simulink model "basic_04_robot"  (R2016a)
settings: Solver=FixedStepAuto  StartTime=0.0  StopTime=inf  FixedStep=0.001  RelTol=1e-3
libraries: Robot_ToolBox x20
settings Model: SimulationMode=external  Creator=Wang Yifan  LastModifiedBy=Wang Yifan
settings OptimizationCC: OptimizeModelRefInitCode=on  LifeSpan=Inf
settings HardwareCC: ProdBitPerLong=64  ProdHWDeviceType=Intel->x86-64 (Linux 64)  TargetBitPerLong=64  TargetBitPerPointer=64  TargetLargestAtomicFloat=Float  TargetIntDivRoundTo=Zero  TargetEndianess=LittleEndian  TargetWordSize=64  TargetHWDeviceType=Intel->x86-64 (Linux 64)  ProdEqTarget=off
settings RTWCC: SystemTargetFile=linux_ert_target.tlc  GenCodeOnly=on  MakeCommand=make_rtw CC=gcc  TemplateMakefile=linux_ert_target.tmf  Description=Linux Embedded Real-Time target  RetainRTWFile=on
settings CodeAppCC: ForceParamTrailComments=on  IgnoreCustomStorageClasses=off  OperatorAnnotations=on  SimulinkDataObjDesc=on  SFDataObjDesc=on  MATLABFcnDesc=on  InsertBlockDesc=on  MATLABSourceComments=on
settings STFCustomTargetCC: CombineOutputUpdateFcns=on  ERTCustomFileBanners=on  SupportContinuousTime=off  SupportNonInlinedSFcns=off  MATLABClassNameForMDSCustomization=Simulink.SoftwareTarget.ERTCustomization  GRTInterface=off  SystemTargetFile=linux_ert_target.tlc
settings ERTTargetCC: ParMdlRefBuildCompliant=off  CompOptLevelCompliant=off  ConcurrentExecutionCompliant=off  ERTFirstTimeCompliant=off  ModelStepFunctionPrototypeControlCompliant=off  CPPClassGenCompliant=off  UseToolchainInfoCompliant=off  ExtMode=on  ExtModeMexArgs='192.168.0.99' 1 17725  ERTSrcFileBannerTemplate=linux_ert_target_code_template.cgt  ERTHdrFileBannerTemplate=linux_ert_target_code_template.cgt  ERTDataSrcFileTemplate=linux_ert_target_code_template.cgt  ERTDataHdrFileTemplate=linux_ert_target_code_template.cgt  ERTCustomFileTemplate=linux_ert_target_generate_main.tlc

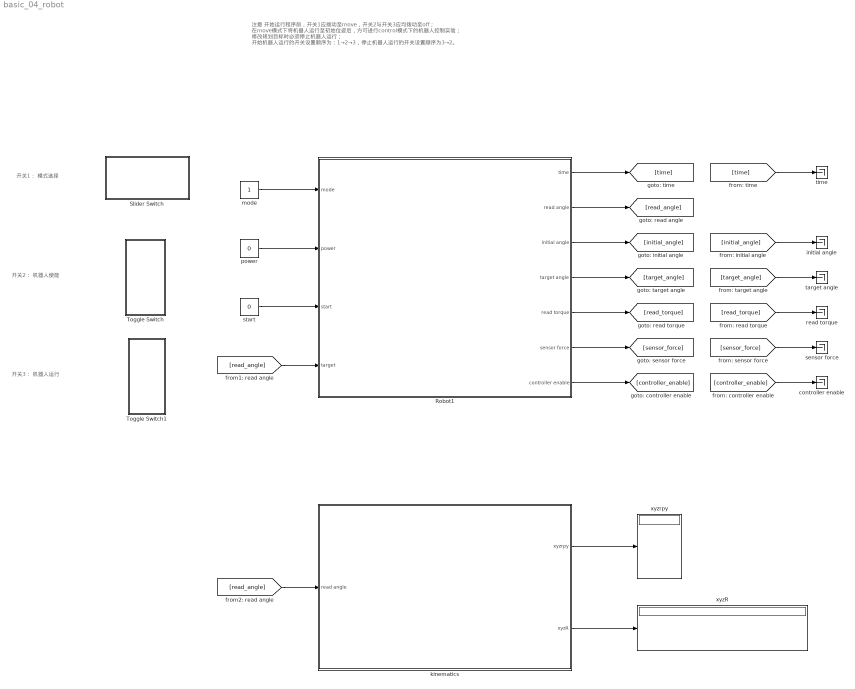
== system basic_04_robot ==
  note: 开关3： 机器人运行
  note: 开关1： 模式选择
  note: 开关2： 机器人使能
  note: 注意
      |
      | 开始运行程序前，开关1应拨动至move，开关2与开关3应均拨动至off；
      | 在move模式下将机器人运行至初始位姿后，方可进行control模式下的机器人控制实验；
      | 修改规划目标时必须停止机器人运行；
      | 开始机器人运行的开关设置顺序为：1→2→3，停止机器人运行的开关设置顺序为3→2。
  Robot1 : Subsystem  mask{move_joint=[0 0 0 0 0 0], joint_1_limit=[-pi/2, pi/2], joint_2_limit=[-pi/2, pi/2], joint_3_limit=[-pi/2, pi/2], joint_4_limit=[-pi/2, pi/2], joint_5_limit=[-pi/2, pi/2], joint_6_limit=[-pi/2, pi/2]}
      mask prompts: joint_1_limit "Joint 1"; joint_2_limit "Joint 2"; joint_3_limit "Joint 3"; joint_4_limit "Joint 4"; joint_5_limit "Joint 5"; joint_6_limit "Joint 6"
      mask DialogControl Container1 Prompt: 目标关节角(rad)
      mask DialogControl Control1 Prompt: e.g. [0 0 0 0 0 0]
      mask DialogControl Container2 Prompt: 关节限位(rad)
      mask DialogControl Control2 Prompt: e.g. [-pi/2, pi/2]
      mask DialogControl Container3 Prompt: 注意：不需要对此模块内部进行修改
  Slider Switch : Subsystem  DialogController=hmiCreateDDGDialog  IsWebBlock=on  mask(MWDashboardBlock){webBlockId=826f4840-ab60-43d7-9b3b-f5102fb9e134, webBlockType=sliderswitch, ShowInLibBrowser=on, ShowInitialText=on, HMISrcModelName=basic_04_robot}
      mask prompts: webBlockId "WebBlock Id"; webBlockType "WebBlock Type"; HMISrcModelName "Source Model"
      mask Help: helpview([docroot '/mapfiles/simulink.map'], 'hmi_slider_switch')
      mask Display:
      | if strcmp(get_param(bdroot(gcb),'BlockDiagramType'), 'library')
      |     image([(matlabroot) '/toolbox/simulink/hmi/icons/SliderSwitch.png']);
      | end
  Toggle Switch : Subsystem  DialogController=hmiCreateDDGDialog  IsWebBlock=on  mask(MWDashboardBlock){webBlockId=da419e04-a9a7-4766-8422-35a2c91d1971, webBlockType=toggleswitch, ShowInLibBrowser=on, ShowInitialText=on, HMISrcModelName=basic_04_robot}
      mask prompts: webBlockId "WebBlock Id"; webBlockType "WebBlock Type"; HMISrcModelName "Source Model"
      mask Help: helpview([docroot '/mapfiles/simulink.map'], 'hmi_toggle_switch')
      mask Display:
      | if strcmp(get_param(bdroot(gcb),'BlockDiagramType'), 'library')
      |     image([(matlabroot) '/toolbox/simulink/hmi/icons/ToggleSwitch.png']);
      | end
  Toggle Switch1 : Subsystem  DialogController=hmiCreateDDGDialog  IsWebBlock=on  mask(MWDashboardBlock){webBlockId=ca3441fb-96d4-41d4-ba82-c21ec3149ad6, webBlockType=toggleswitch, ShowInLibBrowser=on, ShowInitialText=on, HMISrcModelName=basic_04_robot}
      mask prompts: webBlockId "WebBlock Id"; webBlockType "WebBlock Type"; HMISrcModelName "Source Model"
      mask Help: helpview([docroot '/mapfiles/simulink.map'], 'hmi_toggle_switch')
      mask Display:
      | if strcmp(get_param(bdroot(gcb),'BlockDiagramType'), 'library')
      |     image([(matlabroot) '/toolbox/simulink/hmi/icons/ToggleSwitch.png']);
      | end
  controller enable : Terminator
  initial angle : Terminator
  kinematics : Subsystem
  mode : Constant
  power : Constant  Value=0
  read torque : Terminator
  sensor force : Terminator
  start : Constant  Value=0
  target angle : Terminator
  time : Terminator
  xyzR : Display
      settings: Decimation=6
  xyzrpy : Display
      settings: Decimation=6
  wires:
  mode/1 -> Robot1/1(mode)
  power/1 -> Robot1/2(power)
  Robot1/2(read angle) -> [read_angle]
  Robot1/1(time) -> [time]
  Robot1/7(controller enable) -> [controller_enable]
  Robot1/4(target angle) -> [target_angle]
  Robot1/6(sensor force) -> [sensor_force]
  Robot1/3(initial angle) -> [initial_angle]
  start/1 -> Robot1/3(start)
  Robot1/5(read torque) -> [read_torque]
  [time] -> time/1
  [read_angle] -> kinematics/1(read angle)
  [initial_angle] -> initial angle/1
  [target_angle] -> target angle/1
  [read_torque] -> read torque/1
  [sensor_force] -> sensor force/1
  [controller_enable] -> controller enable/1
  kinematics/1(xyzrpy) -> xyzrpy/1
  kinematics/2(xyzR) -> xyzR/1
  [read_angle] -> Robot1/4(target)

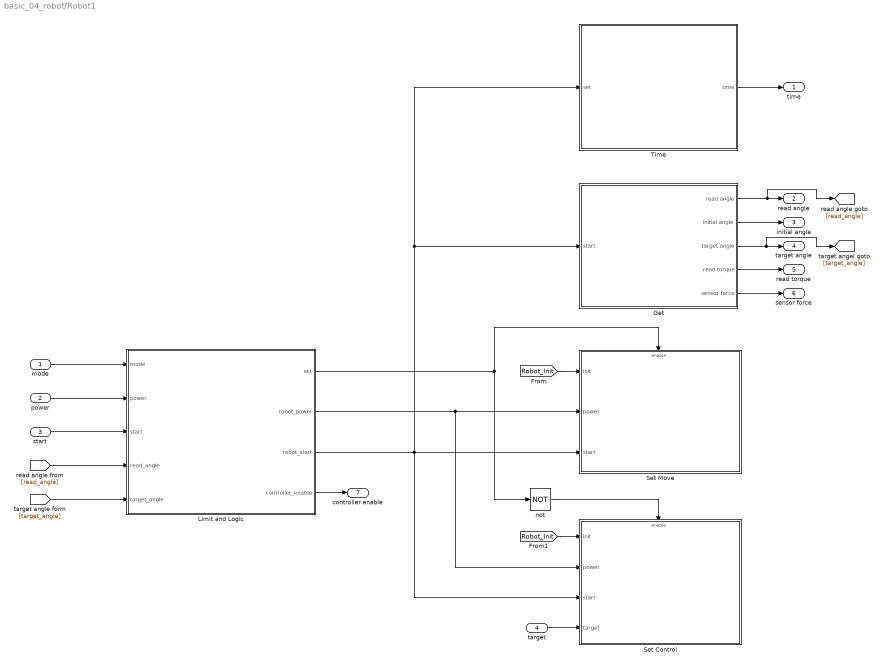
== system basic_04_robot/Robot1 ==
  mode : Inport
  power : Inport  Port=2
  start : Inport  Port=3
  target : Inport  Port=4
  Get : Subsystem
  Limit and Logic : Subsystem
  Set Control : Subsystem  mask(机器人控制模式){mode=Position Mode}
      mask prompts: mode "Control Mode"
      mask TypeOptions mode: Position Mode | Torque Mode | Velocity Mode
  Set Move : Subsystem
  Time : Subsystem
  not : Logic  Operator=NOT  AllPortsSameDT=off  OutDataTypeStr=boolean
  time : Outport
  read angle : Outport  Port=2
  initial angle : Outport  Port=3
  target angle : Outport  Port=4
  read torque : Outport  Port=5
  sensor force : Outport  Port=6
  controller enable : Outport  Port=7
  wires:
  target/1 -> Set Control/4(target)
  Get/1(read angle) -> [read_angle], read angle/1
  Time/1(time) -> time/1
  Get/2(initial angle) -> initial angle/1
  Get/3(target angle) -> [target_angle], target angle/1
  Get/5(sensor force) -> sensor force/1
  Limit and Logic/1(set) -> Set Move/Enable, not/1
  not/1 -> Set Control/Enable
  Limit and Logic/2(robot_power) -> Set Control/2(power), Set Move/2(power)
  Limit and Logic/4(controller_enable) -> controller enable/1
  Limit and Logic/3(robot_start) -> Set Control/3(start), Set Move/3(start), Time/1(set), Get/1(start)
  [Robot_Init] -> Set Move/1(init)
  [Robot_Init] -> Set Control/1(init)
  Get/4(read torque) -> read torque/1
  mode/1 -> Limit and Logic/1(mode)
  power/1 -> Limit and Logic/2(power)
  start/1 -> Limit and Logic/3(start)
  [read_angle] -> Limit and Logic/4(read_angle)
  [target_angle] -> Limit and Logic/5(target_angle)

== system basic_04_robot/Slider Switch ==

== system basic_04_robot/Toggle Switch ==

== system basic_04_robot/Toggle Switch1 ==

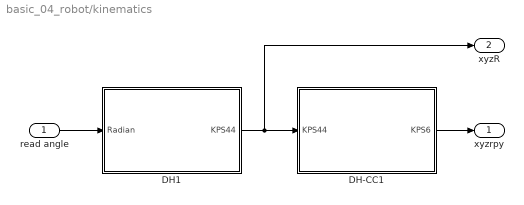
== system basic_04_robot/kinematics ==
  read angle : Inport
  DH-CC1 : MATLAB Function  TreatAsAtomicUnit=on
  DH1 : MATLAB Function  TreatAsAtomicUnit=on
  xyzrpy : Outport
  xyzR : Outport  Port=2
  wires:
  DH1/1(KPS44) -> xyzR/1, DH-CC1/1(KPS44)
  read angle/1 -> DH1/1(Radian)
  DH-CC1/1(KPS6) -> xyzrpy/1

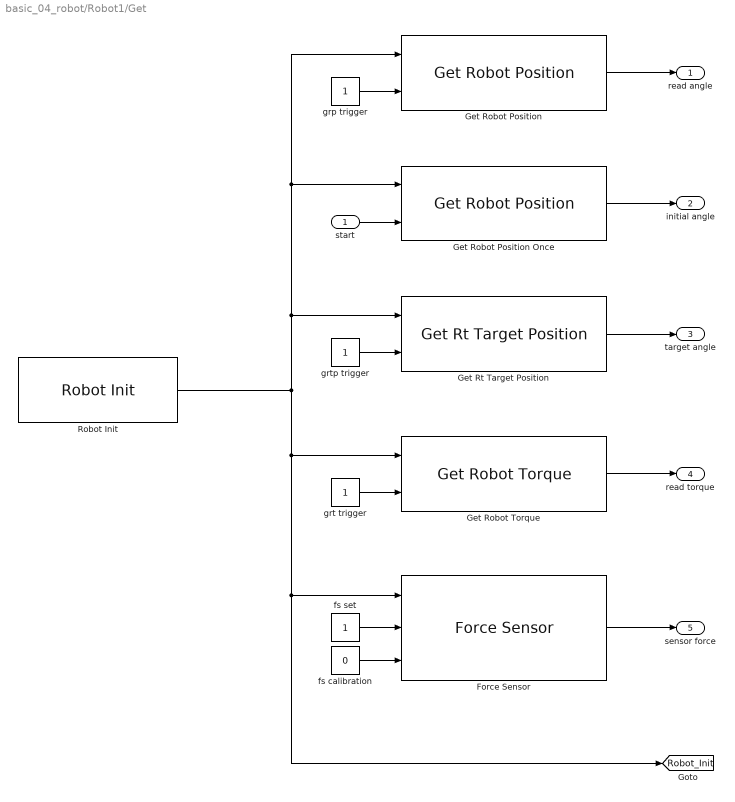
== system basic_04_robot/Robot1/Get ==
  start : Inport
  Force Sensor : Robot_ToolBox/Sensor/Force Sensor  p_robot_index=0  p_torsensor_index=0  p_tool=0  p_wobj=0  p_system_tor_flag=off  p_transform_flag=on
  Get Robot Position : Robot_ToolBox/Robot Interface/Get Robot Position  p_robot_index=0  p_block_index=1  p_read_once=off
  Get Robot Position Once : Robot_ToolBox/Robot Interface/Get Robot Position  p_robot_index=0  p_block_index=0  p_read_once=on
  Get Robot Torque : Robot_ToolBox/Robot Interface/Get Robot Torque  p_robot_index=0  p_block_index=0  p_read_once=off
  Get Rt Target Position : Robot_ToolBox/Robot Interface/Get Rt Target Position  p_robot_index=0  p_block_index=0  p_read_once=off
  Robot Init : Robot_ToolBox/Robot System Tool/Robot Init
  fs calibration : Constant  Value=0
  fs set : Constant
  grp trigger : Constant
  grt trigger : Constant
  grtp trigger : Constant
  read angle : Outport
  initial angle : Outport  Port=2
  target angle : Outport  Port=3
  read torque : Outport  Port=4
  sensor force : Outport  Port=5
  tag scope: Robot_Init=global
  wires:
  Robot Init/1 -> Get Robot Position/1, Get Robot Position Once/1, Get Rt Target Position/1, [Robot_Init], Force Sensor/1, Get Robot Torque/1
  Get Robot Position/1 -> read angle/1
  Get Robot Position Once/1 -> initial angle/1
  Get Rt Target Position/1 -> target angle/1
  Force Sensor/1 -> sensor force/1
  grp trigger/1 -> Get Robot Position/2
  grtp trigger/1 -> Get Rt Target Position/2
  fs set/1 -> Force Sensor/2
  fs calibration/1 -> Force Sensor/3
  start/1 -> Get Robot Position Once/2
  grt trigger/1 -> Get Robot Torque/2
  Get Robot Torque/1 -> read torque/1

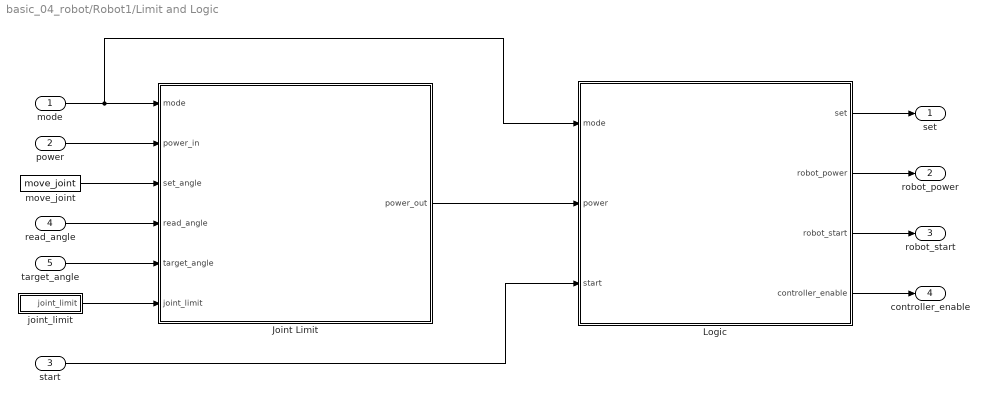
== system basic_04_robot/Robot1/Limit and Logic ==
  mode : Inport
  power : Inport  Port=2
  start : Inport  Port=3
  read_angle : Inport  Port=4
  target_angle : Inport  Port=5
  Joint Limit : MATLAB Function  TreatAsAtomicUnit=on
  Logic : Stateflow chart  TreatAsAtomicUnit=on
  joint_limit : Subsystem
  move_joint : Constant  Value=move_joint
  set : Outport
  robot_power : Outport  Port=2
  robot_start : Outport  Port=3
  controller_enable : Outport  Port=4
  wires:
  Joint Limit/1(power_out) -> Logic/2(power)
  read_angle/1 -> Joint Limit/4(read_angle)
  target_angle/1 -> Joint Limit/5(target_angle)
  mode/1 -> Logic/1(mode), Joint Limit/1(mode)
  power/1 -> Joint Limit/2(power_in)
  start/1 -> Logic/3(start)
  Logic/1(set) -> set/1
  Logic/2(robot_power) -> robot_power/1
  Logic/3(robot_start) -> robot_start/1
  Logic/4(controller_enable) -> controller_enable/1
  move_joint/1 -> Joint Limit/3(set_angle)
  joint_limit/1(joint_limit) -> Joint Limit/6(joint_limit)

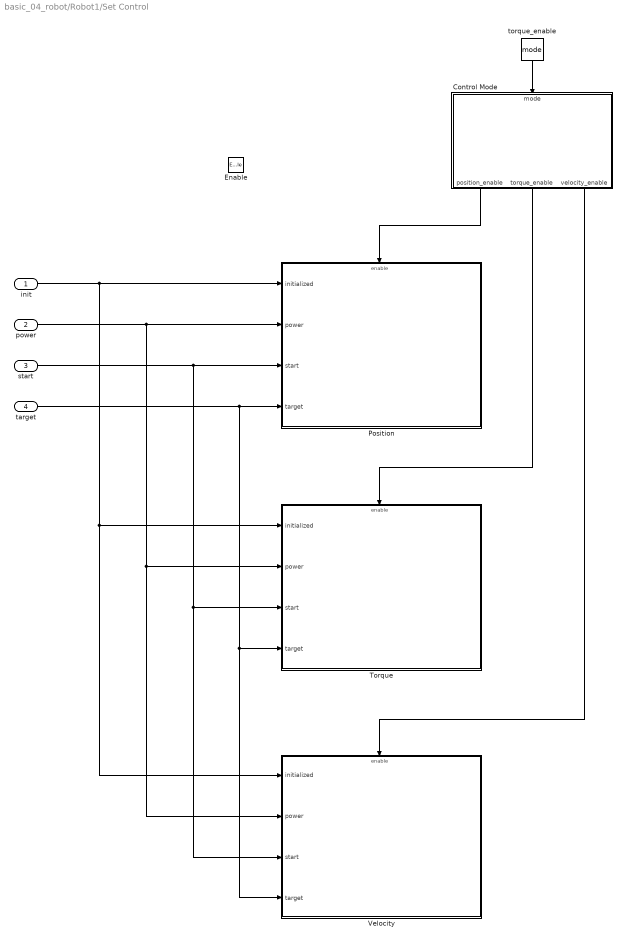
== system basic_04_robot/Robot1/Set Control ==
  init : Inport
  power : Inport  Port=2
  start : Inport  Port=3
  target : Inport  Port=4
  Enable : EnablePort
  Control Mode : Stateflow chart  TreatAsAtomicUnit=on
  Position : Subsystem
  Torque : Subsystem
  Velocity : Subsystem
  torque_enable : Constant  Value=mode
  wires:
  init/1 -> Position/1(initialized), Velocity/1(initialized), Torque/1(initialized)
  power/1 -> Velocity/2(power), Torque/2(power), Position/2(power)
  start/1 -> Velocity/3(start), Torque/3(start), Position/3(start)
  target/1 -> Velocity/4(target), Torque/4(target), Position/4(target)
  Control Mode/1(position_enable) -> Position/Enable
  torque_enable/1 -> Control Mode/1(mode)
  Control Mode/2(torque_enable) -> Torque/Enable
  Control Mode/3(velocity_enable) -> Velocity/Enable

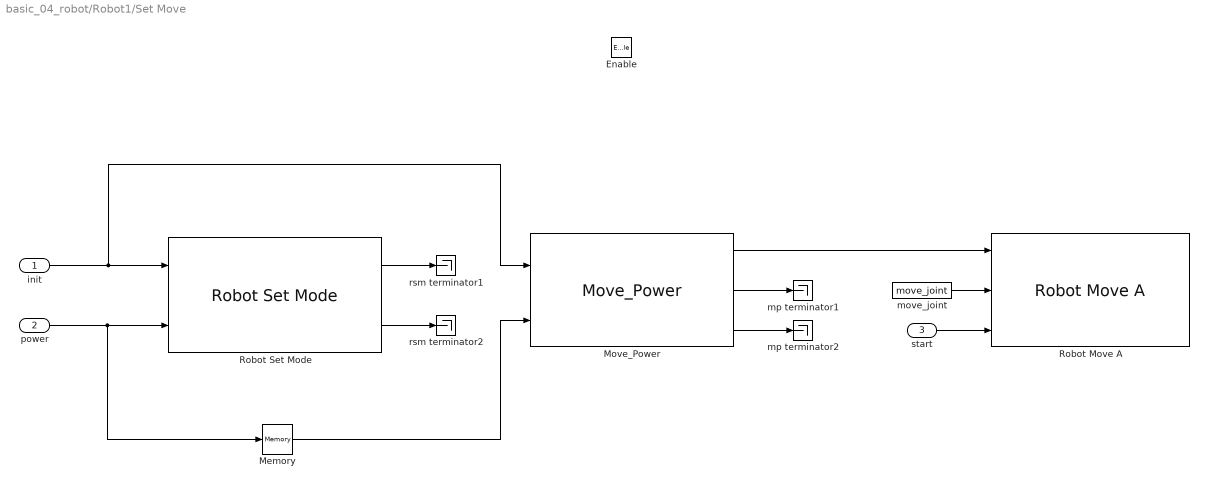
== system basic_04_robot/Robot1/Set Move ==
  init : Inport
  power : Inport  Port=2
  start : Inport  Port=3
  Enable : EnablePort
  Memory : Memory
  Move_Power : Robot_ToolBox/Robot Base Conrtrol/Move_Power  p_robot_index=0  p_block_index=0
      link override S-Function Builder: Parameters=p_robot_index,p_block_index,p_move_thread
  Robot Move A : Robot_ToolBox/Robot Base Conrtrol/Robot Move A  p_robot_index=0  p_block_index=0  p_MoveA_per=[10 10 10 10 10 10]  p_MoveA_per_flag=2  p_zone=0  p_tool=0  p_wobj=0
      link override MoveA: Parameters=p_robot_index,p_block_index,p_MoveA_per,int32(p_MoveA_per_flag),p_zone,p_tool,p_wobj
  Robot Set Mode : Robot_ToolBox/Robot System Tool/Robot Set Mode  p_robot_index=0  p_block_index=0  p_robot_mode=位置模式  p_robot_all=on  p_robot_Axis1=on  p_robot_Axis2=on  p_robot_Axis3=on  p_robot_Axis4=on  p_robot_Axis5=on  p_robot_Axis6=on  p_robot_Axis_add=off
  move_joint : Constant  Value=move_joint
  mp terminator1 : Terminator
  mp terminator2 : Terminator
  rsm terminator1 : Terminator
  rsm terminator2 : Terminator
  wires:
  Move_Power/1 -> Robot Move A/1
  move_joint/1 -> Robot Move A/2
  Move_Power/2 -> mp terminator1/1
  Move_Power/3 -> mp terminator2/1
  start/1 -> Robot Move A/3
  power/1 -> Robot Set Mode/2, Memory/1
  Robot Set Mode/1 -> rsm terminator1/1
  Memory/1 -> Move_Power/2
  Robot Set Mode/2 -> rsm terminator2/1
  init/1 -> Move_Power/1, Robot Set Mode/1

== system basic_04_robot/Robot1/Time ==
  set : Inport
  MATLAB Function : MATLAB Function  TreatAsAtomicUnit=on
  Memory : Memory
  time : Outport
  wires:
  set/1 -> MATLAB Function/1(set)
  MATLAB Function/1(t_out) -> time/1, Memory/1
  Memory/1 -> MATLAB Function/2(t_in)

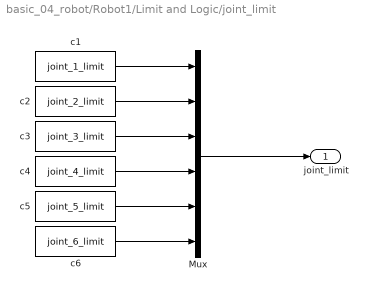
== system basic_04_robot/Robot1/Limit and Logic/joint_limit ==
  Mux : Mux  Inputs=6
  c1 : Constant  Value=joint_1_limit
  c2 : Constant  Value=joint_2_limit
  c3 : Constant  Value=joint_3_limit
  c4 : Constant  Value=joint_4_limit
  c5 : Constant  Value=joint_5_limit
  c6 : Constant  Value=joint_6_limit
  joint_limit : Outport
  wires:
  c1/1 -> Mux/1
  c2/1 -> Mux/2
  c3/1 -> Mux/3
  c4/1 -> Mux/4
  c5/1 -> Mux/5
  c6/1 -> Mux/6
  Mux/1 -> joint_limit/1

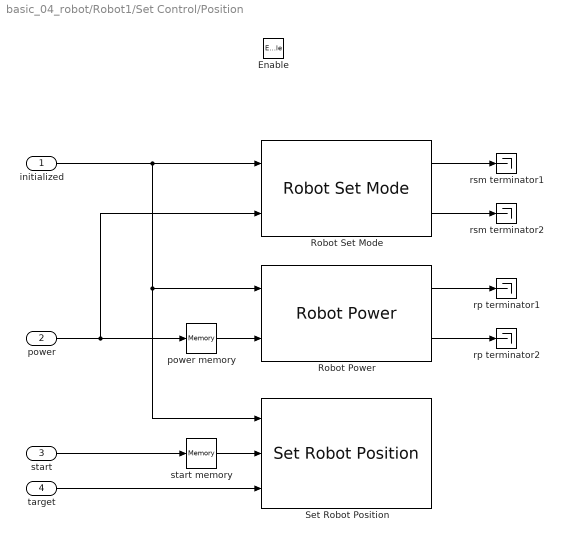
== system basic_04_robot/Robot1/Set Control/Position ==
  initialized : Inport
  power : Inport  Port=2
  start : Inport  Port=3
  target : Inport  Port=4
  Enable : EnablePort
  Robot Power : Robot_ToolBox/Robot System Tool/Robot Power  p_robot_index=0  p_block_index=0  p_robot_all=on  p_robot_Axis1=on  p_robot_Axis2=on  p_robot_Axis3=on  p_robot_Axis4=on  p_robot_Axis5=on  p_robot_Axis6=on  p_robot_Axis_add=off
  Robot Set Mode : Robot_ToolBox/Robot System Tool/Robot Set Mode  p_robot_index=0  p_block_index=0  p_robot_mode=位置模式  p_robot_all=on  p_robot_Axis1=on  p_robot_Axis2=on  p_robot_Axis3=on  p_robot_Axis4=on  p_robot_Axis5=on  p_robot_Axis6=on  p_robot_Axis_add=off
  Set Robot Position : Robot_ToolBox/Robot Interface/Set Robot Position  p_robot_index=0  p_block_index=0  p_read_once=off
  power memory : Memory
  rp terminator1 : Terminator
  rp terminator2 : Terminator
  rsm terminator1 : Terminator
  rsm terminator2 : Terminator
  start memory : Memory
  wires:
  Robot Set Mode/1 -> rsm terminator1/1
  Robot Set Mode/2 -> rsm terminator2/1
  Robot Power/2 -> rp terminator2/1
  initialized/1 -> Robot Set Mode/1, Robot Power/1, Set Robot Position/1
  target/1 -> Set Robot Position/3
  Robot Power/1 -> rp terminator1/1
  power/1 -> power memory/1, Robot Set Mode/2
  start memory/1 -> Set Robot Position/2
  start/1 -> start memory/1
  power memory/1 -> Robot Power/2

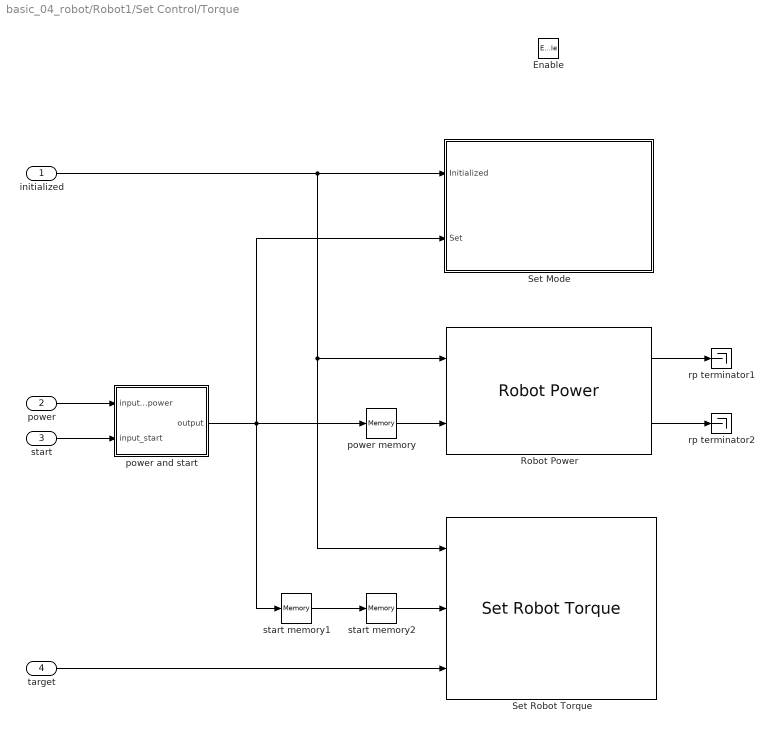
== system basic_04_robot/Robot1/Set Control/Torque ==
  initialized : Inport
  power : Inport  Port=2
  start : Inport  Port=3
  target : Inport  Port=4
  Enable : EnablePort
  Robot Power : Robot_ToolBox/Robot System Tool/Robot Power  p_robot_index=0  p_block_index=0  p_robot_all=off  p_robot_Axis1=off  p_robot_Axis2=off  p_robot_Axis3=off  p_robot_Axis4=off  p_robot_Axis5=off  p_robot_Axis6=on  p_robot_Axis_add=off
  Set Mode : Subsystem
  Set Robot Torque : Robot_ToolBox/Robot Interface/Set Robot Torque  p_robot_index=0  p_block_index=0  p_read_once=off
      link override Set Robot Torque: Parameters=p_robot_index,p_block_index,p_read_once
  power and start : MATLAB Function  TreatAsAtomicUnit=on
  power memory : Memory
  rp terminator1 : Terminator
  rp terminator2 : Terminator
  start memory1 : Memory
  start memory2 : Memory
  wires:
  target/1 -> Set Robot Torque/3
  start memory1/1 -> start memory2/1
  Robot Power/2 -> rp terminator2/1
  Robot Power/1 -> rp terminator1/1
  start memory2/1 -> Set Robot Torque/2
  power memory/1 -> Robot Power/2
  power/1 -> power and start/1(input_power)
  start/1 -> power and start/2(input_start)
  power and start/1(output) -> start memory1/1, Set Mode/2(Set), power memory/1
  initialized/1 -> Robot Power/1, Set Robot Torque/1, Set Mode/1(Initialized)

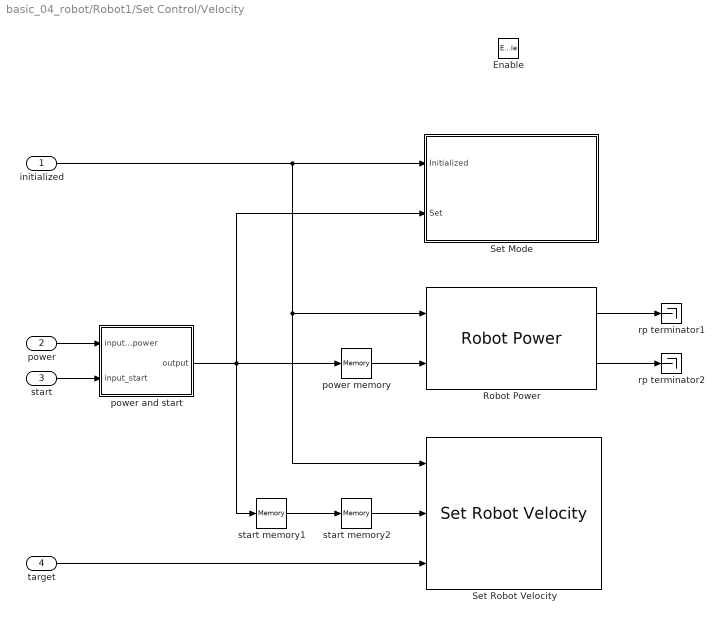
== system basic_04_robot/Robot1/Set Control/Velocity ==
  initialized : Inport
  power : Inport  Port=2
  start : Inport  Port=3
  target : Inport  Port=4
  Enable : EnablePort
  Robot Power : Robot_ToolBox/Robot System Tool/Robot Power  p_robot_index=0  p_block_index=0  p_robot_all=on  p_robot_Axis1=on  p_robot_Axis2=on  p_robot_Axis3=on  p_robot_Axis4=on  p_robot_Axis5=on  p_robot_Axis6=on  p_robot_Axis_add=off
  Set Mode : Subsystem
  Set Robot Velocity : Robot_ToolBox/Robot Interface/Set Robot Velocity  p_robot_index=0  p_block_index=0  p_read_once=off
  power and start : MATLAB Function  TreatAsAtomicUnit=on
  power memory : Memory
  rp terminator1 : Terminator
  rp terminator2 : Terminator
  start memory1 : Memory
  start memory2 : Memory
  wires:
  start memory1/1 -> start memory2/1
  Robot Power/2 -> rp terminator2/1
  Robot Power/1 -> rp terminator1/1
  initialized/1 -> Set Mode/1(Initialized), Robot Power/1, Set Robot Velocity/1
  start memory2/1 -> Set Robot Velocity/2
  power memory/1 -> Robot Power/2
  target/1 -> Set Robot Velocity/3
  power/1 -> power and start/1(input_power)
  start/1 -> power and start/2(input_start)
  power and start/1(output) -> Set Mode/2(Set), power memory/1, start memory1/1

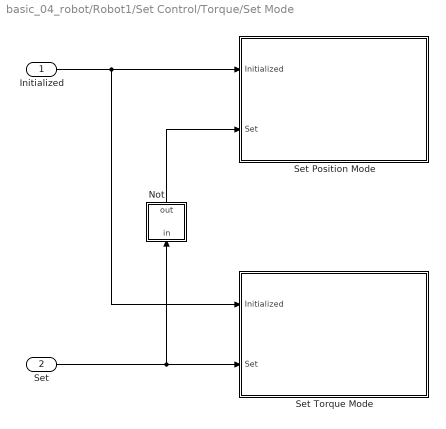
== system basic_04_robot/Robot1/Set Control/Torque/Set Mode ==
  Initialized : Inport
  Set : Inport  Port=2
  Not : MATLAB Function  TreatAsAtomicUnit=on
  Set Position Mode : Subsystem
  Set Torque Mode : Subsystem
  wires:
  Initialized/1 -> Set Position Mode/1(Initialized), Set Torque Mode/1(Initialized)
  Set/1 -> Set Torque Mode/2(Set), Not/1(in)
  Not/1(out) -> Set Position Mode/2(Set)

== system basic_04_robot/Robot1/Set Control/Velocity/Set Mode ==
  Initialized : Inport
  Set : Inport  Port=2
  Not : MATLAB Function  TreatAsAtomicUnit=on
  Set Position Mode : Subsystem
  Set Velocity Mode : Subsystem
  wires:
  Initialized/1 -> Set Position Mode/1(Initialitzed), Set Velocity Mode/1(Initialitzed)
  Set/1 -> Set Velocity Mode/2(Set), Not/1(in)
  Not/1(out) -> Set Position Mode/2(Set)

== system basic_04_robot/Robot1/Set Control/Torque/Set Mode/Set Position Mode ==
  Initialized : Inport
  Set : Inport  Port=2
  Robot Set Mode : Robot_ToolBox/Robot System Tool/Robot Set Mode  p_robot_index=0  p_block_index=0  p_robot_mode=位置模式  p_robot_all=on  p_robot_Axis1=on  p_robot_Axis2=on  p_robot_Axis3=on  p_robot_Axis4=on  p_robot_Axis5=on  p_robot_Axis6=on  p_robot_Axis_add=off
  rsm terminator1 : Terminator
  rsm terminator2 : Terminator
  wires:
  Initialized/1 -> Robot Set Mode/1
  Robot Set Mode/1 -> rsm terminator1/1
  Robot Set Mode/2 -> rsm terminator2/1
  Set/1 -> Robot Set Mode/2

== system basic_04_robot/Robot1/Set Control/Torque/Set Mode/Set Torque Mode ==
  Initialized : Inport
  Set : Inport  Port=2
  Robot Set Mode : Robot_ToolBox/Robot System Tool/Robot Set Mode  p_robot_index=0  p_block_index=0  p_robot_mode=力矩模式  p_robot_all=on  p_robot_Axis1=on  p_robot_Axis2=on  p_robot_Axis3=on  p_robot_Axis4=on  p_robot_Axis5=on  p_robot_Axis6=on  p_robot_Axis_add=off
  rsm terminator1 : Terminator
  rsm terminator2 : Terminator
  wires:
  Robot Set Mode/2 -> rsm terminator2/1
  Robot Set Mode/1 -> rsm terminator1/1
  Set/1 -> Robot Set Mode/2
  Initialized/1 -> Robot Set Mode/1

== system basic_04_robot/Robot1/Set Control/Velocity/Set Mode/Set Position Mode ==
  Initialitzed : Inport
  Set : Inport  Port=2
  Robot Set Mode : Robot_ToolBox/Robot System Tool/Robot Set Mode  p_robot_index=0  p_block_index=0  p_robot_mode=位置模式  p_robot_all=on  p_robot_Axis1=on  p_robot_Axis2=on  p_robot_Axis3=on  p_robot_Axis4=on  p_robot_Axis5=on  p_robot_Axis6=on  p_robot_Axis_add=off
  rsm terminator1 : Terminator
  rsm terminator2 : Terminator
  wires:
  Robot Set Mode/1 -> rsm terminator1/1
  Robot Set Mode/2 -> rsm terminator2/1
  Initialitzed/1 -> Robot Set Mode/1
  Set/1 -> Robot Set Mode/2

== system basic_04_robot/Robot1/Set Control/Velocity/Set Mode/Set Velocity Mode ==
  Initialitzed : Inport
  Set : Inport  Port=2
  Robot Set Mode : Robot_ToolBox/Robot System Tool/Robot Set Mode  p_robot_index=0  p_block_index=0  p_robot_mode=速度模式  p_robot_all=on  p_robot_Axis1=on  p_robot_Axis2=on  p_robot_Axis3=on  p_robot_Axis4=on  p_robot_Axis5=on  p_robot_Axis6=on  p_robot_Axis_add=off
  rsm terminator1 : Terminator
  rsm terminator2 : Terminator
  wires:
  Robot Set Mode/1 -> rsm terminator1/1
  Robot Set Mode/2 -> rsm terminator2/1
  Initialitzed/1 -> Robot Set Mode/1
  Set/1 -> Robot Set Mode/2

== matlab function basic_04_robot/Robot1/Limit and Logic/Joint Limit ==
  data: mode input; power_in input; set_angle input; read_angle input; target_angle input; joint_limit input; power_out output
function power_out = fcn(mode, power_in, set_angle, read_angle, target_angle, joint_limit)

if mode == 1
    for i = 1 : 6
        if (set_angle(i) < joint_limit(2*i-1)) || (set_angle(i) > joint_limit(2*i))
            power_out = 0;
            break;
        else
            power_out = power_in;
            continue;
        end
    end
    
else
    for i = 1 : 6
        if (read_angle(i) < joint_limit(2*i-1)) ...
                || (read_angle(i)> joint_limit(2*i)) ...
                || (target_angle(i) < joint_limit(2*i-1)) ...
                || (target_angle(i)> joint_limit(2*i))
            power_out = 0;
            break;
        else
            power_out = power_in;
            continue;
        end
    end
end
    
end

== stateflow chart basic_04_robot/Robot1/Limit and Logic/Logic ==
  state init
    entry:
    robot_power = 0;
    robot_start = 0;
    controller_enable = 0;
  state move
    entry: set = 1;
    state move_power_on
      entry: robot_power = 1;
      state robot_start_on
        entry:
        robot_start = 1;
        controller_enable = 0;
      state robot_start_off
        entry:
        robot_start = 0;
        controller_enable = 0;
      (default) -> (junction 90)
      (junction 90) -> move.move_power_on.robot_start_off [order 2] : [start == 0]
      (junction 90) -> move.move_power_on.robot_start_on [order 1] : [start == 1]
      move.move_power_on.robot_start_on -> move.move_power_on.robot_start_off : [start == 0]
      move.move_power_on.robot_start_off -> move.move_power_on.robot_start_on : [start == 1]
    state move_power_off
      entry: robot_power = 0;
      state robot_start_off
        entry:
        robot_start = 0;
        controller_enable = 0;
      (default) -> move.move_power_off.robot_start_off
    (default) -> (junction 40)
    (junction 40) -> move_power_off [order 2] : [power == 0]
    (junction 40) -> move_power_on [order 1] : [power == 1]
    move_power_on -> move_power_off : [power == 0]
    move_power_off -> move_power_on : [power == 1 & start == 0]
  state control
    entry: set = 0;
    state control_power_on
      entry: robot_power = 1;
      state robot_start_off
        entry:
        robot_start = 0;
        controller_enable = 0;
      state robot_start_on
        entry:
        robot_start = 1;
        controller_enable = 1;
      (default) -> (junction 73)
      (junction 73) -> control.control_power_on.robot_start_on [order 1] : [start == 1]
      (junction 73) -> control.control_power_on.robot_start_off [order 2] : [start == 0]
      control.control_power_on.robot_start_on -> control.control_power_on.robot_start_off : [start == 0]
      control.control_power_on.robot_start_off -> control.control_power_on.robot_start_on : [start == 1]
    state control_power_off
      entry: robot_power = 0;
      state robot_start_off
        entry:
        robot_start = 0;
        controller_enable = 0;
      (default) -> control.control_power_off.robot_start_off
    (default) -> (junction 50)
    (junction 50) -> control_power_on [order 1] : [power == 1]
    (junction 50) -> control_power_off [order 2] : [power == 0]
    control_power_on -> control_power_off : [power == 0]
    control_power_off -> control_power_on : [power == 1 & start == 0]
  (default) -> (junction 81)
  (junction 81) -> init [order 2] : [power == 1 | start ==1]
  init -> (junction 81)
  (junction 81) -> (junction 32) [order 1] : [power == 0 & start ==0]
  (junction 32) -> control [order 2] : [mode == 0]
  (junction 32) -> move [order 1] : [mode == 1]
  move -> control : [mode == 0 & power == 0]
  control -> move : [mode == 1 & power == 0]
  data: mode input; power input; start input; set output; robot_power output; robot_start output; controller_enable output

== stateflow chart basic_04_robot/Robot1/Set Control/Control Mode ==
  state Init
    entry:
    position_enable = 1;
    torque_enable = 0;
    velocity_enable = 0;
  state Position
    entry:
    position_enable = 1;
    torque_enable = 0;
    velocity_enable = 0;
  state Torque
    entry:
    position_enable = 0;
    torque_enable = 1;
    velocity_enable = 0;
  state Velocity
    entry:
    position_enable = 0;
    torque_enable = 0;
    velocity_enable = 1;
  (default) -> Init
  Init -> (junction 6)
  (junction 6) -> Velocity [order 3] : [mode == 3]
  (junction 6) -> Position [order 1] : [mode == 1]
  (junction 6) -> Torque [order 2] : [mode == 2]
  data: mode input; position_enable output; torque_enable output; velocity_enable output

== matlab function basic_04_robot/Robot1/Set Control/Torque/Set Mode/Not ==
  data: in input; out output
function out = fcn(in)

if in == 0
    out = 1;
else
    out = 0;
end

end

== matlab function basic_04_robot/Robot1/Set Control/Torque/power and start ==
  data: input_power input; output output; input_start input
function output  = fcn(input_power, input_start)

if (input_power == 1) && (input_start == 1)
    output = 1;
else
    output = 0;
end

end

== matlab function basic_04_robot/Robot1/Set Control/Velocity/Set Mode/Not ==
  data: in input; out output
function out = fcn(in)

if in == 0
    out = 1;
else
    out = 0;
end

end

== matlab function basic_04_robot/Robot1/Set Control/Velocity/power and start ==
  data: input_power input; output output; input_start input
function output  = fcn(input_power, input_start)

if (input_power == 1) && (input_start == 1)
    output = 1;
else
    output = 0;
end

end

== matlab function basic_04_robot/Robot1/Time/MATLAB Function ==
  data: set input; t_out output; t_in input
function t_out = timer(set, t_in)

persistent flag;
if isempty(flag)
    flag = 0;
end

if set == 1
    t_out = t_in + 0.001;
else
    t_out = 0;
end

end

== matlab function basic_04_robot/kinematics/DH-CC1 ==
  data: KPS44 input; KPS6 output
function KPS6  = FK(KPS44)
%% parameter
rpy = zeros(1,3);
eps = 0.000001;
%% input 
T=[1 0 0 0;0 1 0 0; 0 0 1 0];
G=KPS44;
H =T * ( G * [0;0;0;1]);
%%
rpy(2) = atan2(-KPS44(3,1),sqrt(KPS44(1,1)*KPS44(1,1)+KPS44(2,1)*KPS44(2,1)));
if (abs(abs(rpy(2)) - pi / 2.0) < eps)
	if (rpy(2) > 0) 
        rpy(2) = pi / 2.0;
        rpy(3) = 0.0;
        rpy(1) = atan2(KPS44(1,2),KPS44(2,2));
    else
    rpy(2) = -pi / 2.0;
	rpy(3) = 0.0;
	rpy(1) = -atan2(KPS44(1,2), KPS44(2,2));
	end
else
	cp = cos(rpy(2));
	rpy(3) = atan2(KPS44(2,1)/cp,KPS44(1,1)/cp);
	rpy(1) = atan2(KPS44(3,2)/cp, KPS44(3,3)/cp);
end
KPS6 = [H' rpy]; 
end

== matlab function basic_04_robot/kinematics/DH1 ==
  data: Radian input; KPS44 output
function KPS44  = FK(Radian)

%% input 
theta1 = Radian(1);
theta2 = Radian(2);
theta3 = Radian(3);
theta4 = Radian(4);
theta5 = Radian(5);
theta6 = Radian(6);
offset2 = -pi/2; offset3 =0;
Q=[theta1;theta2+offset2;theta3+offset3;theta4;theta5;theta6];
%% D-H parameters 
%XB4
d1=342;a1=40;a2=275;a3=25;d4=280;dt=73;d3=0;
%XB7
% d1=380;a1=30;a2=340;a3=35;d4=345;dt=87;d3=0;

Tbase = [1 0 0 0;
        0 1 0 0;
        0 0 1 d1;
        0 0 0 1];
Ttool = [1 0 0 0;
        0 1 0 0;
        0 0 1 dt;
        0 0 0 1];
%% output
II = zeros(4,4);

%% T1~T6
s1=sin(Q(1));s2=sin(Q(2));s3=sin(Q(3));s4=sin(Q(4));s5=sin(Q(5));s6=sin(Q(6));
c1=cos(Q(1));c2=cos(Q(2));c3=cos(Q(3));c4=cos(Q(4));c5=cos(Q(5));c6=cos(Q(6));

t14 = a1*c1 + a3*(c1*c2*c3 - c1*s2*s3) - d3*s1 - d4*(c1*c2*s3 + c1*c3*s2) + a2*c1*c2;
t24 = a1*s1 + c1*d3 + a3*(c2*c3*s1 - s1*s2*s3) - d4*(c2*s1*s3 + c3*s1*s2) + a2*c2*s1;
t34 =-a2*s2 - a3*(c2*s3 + c3*s2) - d4*(c2*c3 - s2*s3);

t11 =s6*(c4*s1 - s4*(c1*c2*c3 - c1*s2*s3)) - c6*(s5*(c1*c2*s3 + c1*c3*s2) - c5*(s1*s4 + c4*(c1*c2*c3 - c1*s2*s3)));
t21 = - c6*(s5*(c2*s1*s3 + c3*s1*s2) + c5*(c1*s4 - c4*(c2*c3*s1 - s1*s2*s3))) - s6*(c1*c4 + s4*(c2*c3*s1 - s1*s2*s3));
t31 = s4*s6*(c2*s3 + c3*s2) - c6*(s5*(c2*c3 - s2*s3) + c4*c5*(c2*s3 + c3*s2));
t12 = s6*(s5*(c1*c2*s3 + c1*c3*s2) - c5*(s1*s4 + c4*(c1*c2*c3 - c1*s2*s3))) + c6*(c4*s1 - s4*(c1*c2*c3 - c1*s2*s3));
t22 =s6*(s5*(c2*s1*s3 + c3*s1*s2) + c5*(c1*s4 - c4*(c2*c3*s1 - s1*s2*s3))) - c6*(c1*c4 + s4*(c2*c3*s1 - s1*s2*s3));
t32 =s6*(s5*(c2*c3 - s2*s3) + c4*c5*(c2*s3 + c3*s2)) + c6*s4*(c2*s3 + c3*s2);
t13= - c5*(c1*c2*s3 + c1*c3*s2) - s5*(s1*s4 + c4*(c1*c2*c3 - c1*s2*s3));
t23 = s5*(c1*s4 - c4*(c2*c3*s1 - s1*s2*s3)) - c5*(c2*s1*s3 + c3*s1*s2);
t33 = c4*s5*(c2*s3 + c3*s2) - c5*(c2*c3 - s2*s3);


II = [t11 t12 t13 t14;
         t21 t22 t23 t24;
         t31 t32 t33 t34;
         0 0 0 1];
     
KPS44 = Tbase*II*Ttool;

end
